simulink model "SMC"  (R2026a)
settings: Solver=VariableStepAuto  StopTime=inf
model workspace (MAT data in the model file):
  reach_rate = [3; 3; 3; 4; 2]
undefined symbols (not defined in the file): force, torque
libraries: ros2lib x4, slctrl_smc x1
settings Model: Creator=hashaam1217  LastModifiedBy=root

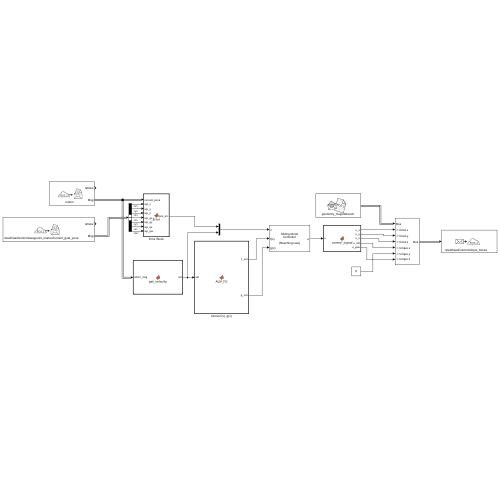
[thumbnail: Simulink's stored preview of the top-level diagram]
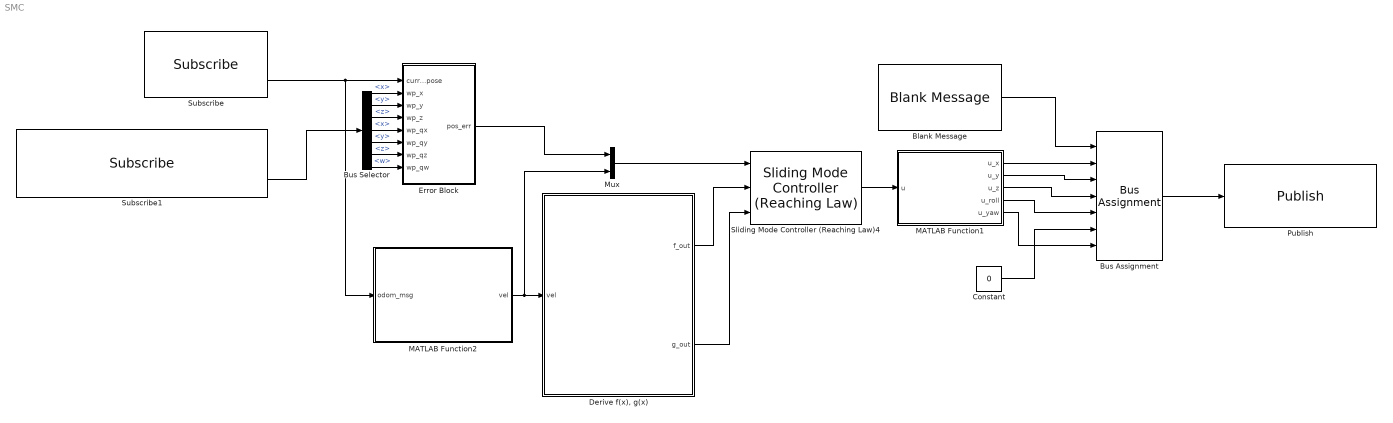
== system SMC ==
  Blank Message : ros2lib/Blank Message  messageClass=Message  entityType=geometry_msgs/Wrench  messageType=geometry_msgs/Wrench  SampleTime=inf
  Bus Assignment : BusAssignment  AssignedSignals=force.x,force.y,force.z,torque.x,torque.y,torque.z
  Bus Selector : BusSelector  OutputSignals=position.x,position.y,position.z,orientation.x,orientation.y,orientation.z,orientation.w
  Constant : Constant  Value=0
  "Derive f(x), g(x)" : MATLAB Function  TreatAsAtomicUnit=on
  Error Block : MATLAB Function  TreatAsAtomicUnit=on
  MATLAB Function1 : MATLAB Function  TreatAsAtomicUnit=on
  MATLAB Function2 : MATLAB Function  TreatAsAtomicUnit=on
  Mux : Mux  Inputs=2
  Publish : ros2lib/Publish  topicSource=Specify your own  topic=/steelhead/controls/input_forces  messageType=geometry_msgs/Wrench  QOSHistory=Keep last  QOSDepth=10  QOSReliability=Reliable  QOSDurability=Volatile  QOSDeadline=Inf  QOSLifespan=Inf  QOSLiveliness=Automatic  QOSLeaseDuration=Inf  QOSAvoidROSNamespaceConventions=off
  Sliding Mode Controller (Reaching Law)4 : slctrl_smc/Sliding Mode Controller (Reaching Law)  TaskMode=Regulation Mode  SlidingMatrix=[5*eye(5); eye(5)]  EnableTrackingDerivative=off  EnableSwitchingFunction=off  ReachingLaw=Exponential  ReachingRate=3  ControlGain=2  PowerRate=0.01  BoundaryLayer=Saturation  ZeroCross=off  Phi=0.05
  Subscribe : ros2lib/Subscribe  topicSource=Select from ROS network  topic=/odom  messageType=nav_msgs/Odometry  sampleTime=0.02  QOSHistory=Keep all  QOSDepth=10  QOSReliability=Reliable  QOSDurability=Volatile  QOSDeadline=Inf  QOSLifespan=Inf  QOSLiveliness=Automatic  QOSLeaseDuration=Inf  QOSAvoidROSNamespaceConventions=off
  Subscribe1 : ros2lib/Subscribe  topicSource=Specify your own  topic=/steelhead/controls/waypoint_marker/current_goal_pose  messageType=geometry_msgs/Pose  sampleTime=-1  QOSHistory=Keep last  QOSDepth=10  QOSReliability=Reliable  QOSDurability=Volatile  QOSDeadline=Inf  QOSLifespan=Inf  QOSLiveliness=Automatic  QOSLeaseDuration=Inf  QOSAvoidROSNamespaceConventions=off
  wires:
  Subscribe/2 -> Error Block/1(current_pose), MATLAB Function2/1(odom_msg)
  Bus Assignment/1 -> Publish/1
  Constant/1 -> Bus Assignment/6
  Sliding Mode Controller (Reaching Law)4/1 -> MATLAB Function1/1(u)
  MATLAB Function1/1(u_x) -> Bus Assignment/2
  MATLAB Function1/2(u_y) -> Bus Assignment/3
  MATLAB Function1/3(u_z) -> Bus Assignment/4
  MATLAB Function1/5(u_yaw) -> Bus Assignment/7
  MATLAB Function2/1(vel) -> Mux/2, "Derive f(x), g(x)"/1(vel)
  "Derive f(x), g(x)"/1(f_out) -> Sliding Mode Controller (Reaching Law)4/2
  "Derive f(x), g(x)"/2(g_out) -> Sliding Mode Controller (Reaching Law)4/3
  Error Block/1(pos_err) -> Mux/1
  Mux/1 -> Sliding Mode Controller (Reaching Law)4/1
  Blank Message/1 -> Bus Assignment/1
  MATLAB Function1/4(u_roll) -> Bus Assignment/5
  Subscribe1/2 -> Bus Selector/1
  Bus Selector/1 -> Error Block/2(wp_x)  "<x>"
  Bus Selector/2 -> Error Block/3(wp_y)  "<y>"
  Bus Selector/3 -> Error Block/4(wp_z)  "<z>"
  Bus Selector/4 -> Error Block/5(wp_qx)  "<x>"
  Bus Selector/5 -> Error Block/6(wp_qy)  "<y>"
  Bus Selector/6 -> Error Block/7(wp_qz)  "<z>"
  Bus Selector/7 -> Error Block/8(wp_qw)  "<w>"

== matlab function SMC/Error Block ==
  data: current_pose input; pos_err output; wp_x input; wp_y input; wp_z input; wp_qx input; wp_qy input; wp_qz input; wp_qw input
function pos_err = Error(current_pose, wp_x, wp_y, wp_z, wp_qx, wp_qy, wp_qz, wp_qw)

      current_position    = current_pose.pose.pose.position;
      current_orientation = current_pose.pose.pose.orientation;

      dx = wp_x - current_position.x;
      dy = wp_y - current_position.y;
      dz = wp_z - current_position.z;

      qx = current_orientation.x;
      qy = current_orientation.y;
      qz = current_orientation.z;
      qw = current_orientation.w;

      R11 = 1 - 2*(qy^2 + qz^2);
      R12 = 2*(qx*qy + qw*qz);
      R13 = 2*(qx*qz - qw*qy);
      R21 = 2*(qx*qy - qw*qz);
      R22 = 1 - 2*(qx^2 + qz^2);
      R23 = 2*(qy*qz + qw*qx);
      R31 = 2*(qx*qz + qw*qy);
      R32 = 2*(qy*qz - qw*qx);
      R33 = 1 - 2*(qx^2 + qy^2);

      err_surge = R11*dx + R12*dy + R13*dz;
      err_sway  = R21*dx + R22*dy + R23*dz;
      err_heave = R31*dx + R32*dy + R33*dz;

      current_yaw  = atan2(2*(qw*qz + qx*qy), 1 - 2*(qy^2 + qz^2));
      current_roll = atan2(2*(qw*qx + qy*qz), 1 - 2*(qx^2 + qy^2));
      desired_yaw  = atan2(2*(wp_qw*wp_qz + wp_qx*wp_qy), 1 - 2*(wp_qy^2 + wp_qz^2));

      err_roll = mod(-current_roll + pi, 2*pi) - pi;
      err_yaw  = mod((desired_yaw - current_yaw) + pi, 2*pi) - pi;

      pos_err = [err_surge; err_sway; err_heave; err_roll; err_yaw];
  end

== matlab function SMC/MATLAB Function1 ==
  data: u input; u_x output; u_y output; u_z output; u_roll output; u_yaw output
function [u_x, u_y, u_z, u_roll, u_yaw] = control_signal(u)

u_x = u(1);
u_y = u(2);
u_z = u(3);
u_roll = u(4);
u_yaw = u(5);

== matlab function SMC/MATLAB Function2 ==
  data: odom_msg input; vel output
function vel  = get_velocity(odom_msg)

    vel_x   = odom_msg.twist.twist.linear.x;
    vel_y   = odom_msg.twist.twist.linear.y;
    vel_z   = odom_msg.twist.twist.linear.z;
    vel_roll = odom_msg.twist.twist.angular.x;
    vel_yaw = odom_msg.twist.twist.angular.z;

    vel = [vel_x; vel_y; vel_z; vel_roll; vel_yaw];

end

== matlab function SMC/Derive f(x), g(x) ==
  data: f_out output; vel input; g_out output
function [f_out, g_out] = AUV_FG(vel)

% INPUT:
%   vel = [u; v; w; p; r]  (5x1, body frame velocities from /odom twist)
%         u = surge velocity (x)
%         v = sway velocity  (y)
%         w = heave velocity (z)
%         p = roll rate
%         r = yaw rate
%
% OUTPUTS:
%   f_out = 10x1  (system drift — what AUV does with no thrusters)
%   g_out = 10x5  (control influence — how thruster force affects state)

% PARAMETERS FROM URDF:
mass = 11.2703688048829;
Ixx  = 0.060252345626549;
Izz  = 0.127878964636527;

% PARAMETERS FROM SDF: (scalingAddedMass = 0.01)
Xu_dot = 0.01 * 5.579266667;    
Yv_dot = 0.01 * 15.09083333;   
Zw_dot = 0.01 * 30.55093333;   
Kp_dot = 0.01 * 7.2955698;      
Nr_dot = 0.01 * 16.14743877;     

% MASS MATRIX: (5x5 diagonal)
M = diag([mass+Xu_dot; ...
          mass+Yv_dot; ...
          mass+Zw_dot; ...
          Ixx+Kp_dot; ...
          Izz+Nr_dot]);

M_inv = inv(M);


% DAMPING MATRIX: (5x5 diagonal, dependent on velocity)
u = vel(1);   % surge velocity
v = vel(2);   % sway velocity
w = vel(3);   % heave velocity
p = vel(4);   % roll rate
r = vel(5);   % yaw rate

% linear damping coefficients
Xu = -0.2229119791;      
Yv = -1.105547605;       
Zw = -0.2472084207;      
Kp = -0.02229119791;    
Nr = -0.02472084207;     

% quadratic damping coefficients
Xuu = -59.75066625;     
Yvv = -71.13459739;     
Zww = -67.099009;       
Kpp = -5.975066625;     
Nrr = -6.7099009; 

D = -diag([Xu + Xuu*abs(u);    
           Yv + Yvv*abs(v);    
           Zw + Zww*abs(w);   
           Kp + Kpp*abs(p);   
           Nr + Nrr*abs(r)]);

restoring = zeros(5,1);

f_out = [vel; M_inv * (-D * vel - restoring)];
g_out = [zeros(5,5); M_inv];
